simulink model "sgMdl_IO3xx_40_A2B_Loopback"  (R2024b)
settings: Solver=FixedStepAuto  StartTime=0.0  StopTime=inf  RelTol=1e-3  EnableMultiTasking=on
undefined symbols (not defined in the file): c, d, IO3xx, Pull, pull, up
libraries: speedgoatlib_a2b x6, simulink x3, speedgoatlib_interrupt x1, speedgoatlib_fpga x1
Description:
  | IO3xx A2B - Loopback
settings Model: ModifiedByFormat=Speedgoat  SimulationMode=external  ExtModeTrigDuration=100000  Creator=Speedgoat  LastModifiedBy=Speedgoat
settings SolverCC: ConcurrentTasks=on  AlgebraicLoopSolver=TrustRegion  PositivePriorityOrder=on  InsertRTBMode=Never (minimum delay)
settings DataIOCC: SaveFormat=Array  SaveState=on  SignalLoggingName=logsOut
settings OptimizationCC: BlockReduction=off  BooleanDataType=off  OptimizeBlockIOStorage=off  BufferReuse=off  GlobalBufferReuse=off  ExpressionFolding=off  LocalBlockOutputs=off  InitFltsAndDblsToZero=on  OptimizeDataStoreBuffers=off  BusAssignmentInplaceUpdate=off
settings DebuggingCC: SaveWithParameterizedLinksMsg=none  CheckExecutionContextPreStartOutputMsg=on  SignalResolutionControl=TryResolveAllWithWarning  TasksWithSamePriorityMsg=none  UnconnectedInputMsg=warning  UnconnectedOutputMsg=warning  UnconnectedLineMsg=warning  SFUnexpectedBacktrackingDiag=warning  SFNoUnconditionalDefaultTransitionDiag=warning  SFExecutionAtInitializationDiag=none  ArithmeticOperatorsInVariantConditions=warning
settings HardwareCC: ProdBitPerLong=64  ProdLongLongMode=on  ProdHWDeviceType=Intel->x86-64 (Linux 64)
settings ModelReferenceCC: EnableRefExpFcnMdlSchedulingChecks=on
settings SFSimCC: SimUseLocalCustomCode=off  SimTargetLang=C++
settings RTWCC: Description=Speedgoat Real-Time Target Machine  SystemTargetFile=speedgoat.tlc  TemplateMakefile=slrealtime_default_tmf  PostCodeGenCommand=sg.model.build.makeCfg(bdroot, buildInfo);  RTWUseLocalCustomCode=off  Toolchain=Simulink Real-Time Toolchain  BuildConfiguration=Faster Runs  TargetLang=C++  GPUComputeCapability=3.5  DLArmComputeVersion=19.05
settings CodeAppCC: StateflowObjectComments=on
settings SimulinkRealTimeTargetCC: SubcomponentCodeInterfacePackaging=Reusable function  MATLABClassNameForMDSCustomization=Simulink.SoftwareTarget.GRTCustomization  InstructionSetFMA=off  LogToMDFFile=off  SLRTFileLogMaxRuns=10  UseGCCFastMath=on
settings ConfigComp: CovMetricSettings=dw  CovSaveCumulativeToWorkspaceVar=on  CovSaveSingleToWorkspaceVar=on  CovExternalEMLEnable=off  CovSFcnEnable=off  CovBoundaryAbsTol=1.0e-5

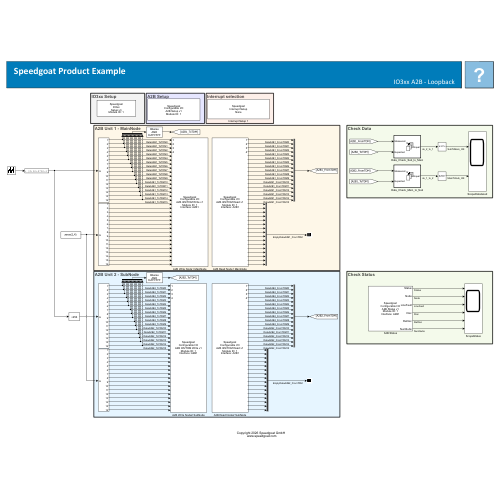
[thumbnail: Simulink's stored preview of the top-level diagram]
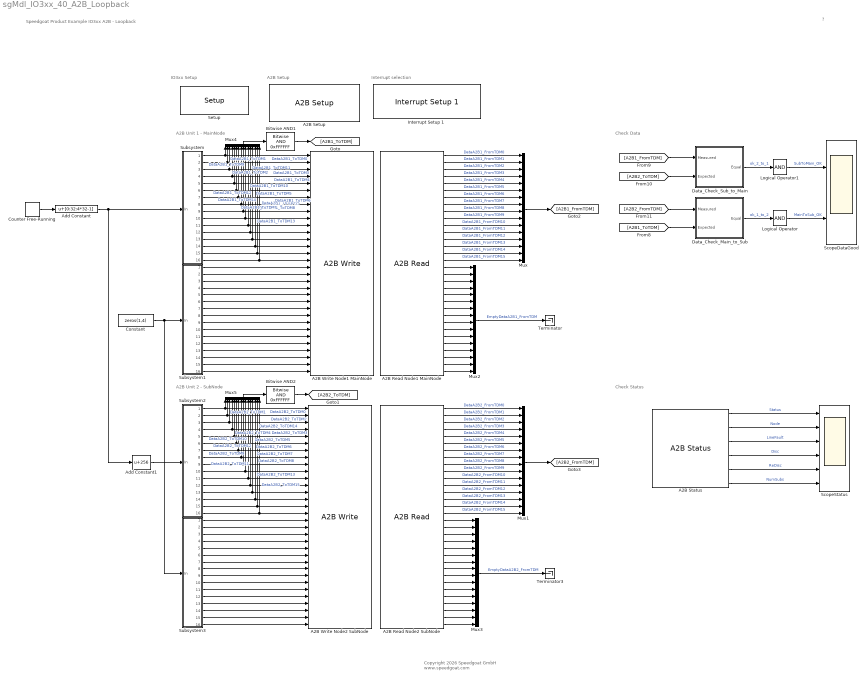
== system sgMdl_IO3xx_40_A2B_Loopback ==
  note: Interrupt selection
  note: A2B Setup
  note: IO3xx Setup
  note: A2B Unit 1 - MainNode
  note: A2B Unit 2 - SubNode
  note: Check Data
  note: Check Status
  note: Speedgoat Product Example
      | IO3xx A2B - Loopback
  note: ?
  note: Copyright 2026 Speedgoat GmbH
      |  www.speedgoat.com
  A2B Read Node1 MainNode : speedgoatlib_a2b/A2B Read   parModuleId=1  parPosition=A2B1  parFrameSize=4  parTdmMode=16  parTdmSize=32  parDataSize=24  parSampleTime=-1
  A2B Read Node2 SubNode : speedgoatlib_a2b/A2B Read   parModuleId=1  parPosition=A2B2  parFrameSize=4  parTdmMode=16  parTdmSize=32  parDataSize=24  parSampleTime=-1
  "A2B Setup " : speedgoatlib_a2b/A2B Setup   parModuleId=1  parPosition=1  parTdmChSize=[32 32 16 16]  parTdmMode=[16 16 0 0]  parA2BdownSlotSize=[24 0 0 0]  parA2BupSlotSize=[24 0 16 16]  parChecksum=2BC6806296FB9E7142791A9417BDFF8D,3D277645F3D52ECCF21C75D98A92E88D,c,d'  parMode1=Main Node  parMode2=Subordinate Node  parMode3=Disabled  parMode4=Disabled  parAudioClock=48kHz  parFrameSize=4  parSampleTime=4/48e3  parNetworkConfig1=''  parNodeConfig1=''  parNetworkConfig2=''  parNodeConfig2=''  parNetworkConfig3=''  parNodeConfig3=''  parNetworkConfig4=''  parNodeConfig4=''
  A2B Status : speedgoatlib_a2b/A2B Status   parModuleId=1  parChipId=A2B1  parEnPwr=on  parEnDiscovery=on  parEnBusDiscovery=on  parEnSlaveNodes=on  parSampleTime=50*4/48e3
  A2B Write Node1 MainNode : speedgoatlib_a2b/A2B Write   parModuleId=1  parPosition=A2B1  parFrameSize=4  parTdmMode=16  parTdmSize=32  parDataSize=24  parSampleTime=-1
  A2B Write Node2 SubNode : speedgoatlib_a2b/A2B Write   parModuleId=1  parPosition=A2B2  parFrameSize=4  parTdmMode=16  parTdmSize=32  parDataSize=24  parSampleTime=-1
  Add Constant : Bias  Bias=[0:32:4*32-1]  SaturateOnIntegerOverflow=off
  Add Constant1 : Bias  Bias=256  SaturateOnIntegerOverflow=off
  Bitwise AND1 : simulink/Logic and Bit Operations/Bitwise Operator  logicop=AND  UseBitMask=on  BitMask=0xFFFFFF  BitMaskRealWorld=Stored Integer
      settings: LibrarySourceBlock=|
      | simulink/Quick Insert/Logic and Bit
      | Operations/Bitwise AND
  Bitwise AND2 : simulink/Logic and Bit Operations/Bitwise Operator  logicop=AND  UseBitMask=on  BitMask=0xFFFFFF  BitMaskRealWorld=Stored Integer
      settings: LibrarySourceBlock=|
      | simulink/Quick Insert/Logic and Bit
      | Operations/Bitwise AND
  Constant : Constant  Value=zeros(1,4)  OutDataTypeStr=uint32
  Counter Free-Running : simulink/Sources/Counter Free-Running  NumBits=32  tsamp=-1
  Data_Check_Main_to_Sub : Subsystem  TreatAsAtomicUnit=on
  Data_Check_Sub_to_Main : Subsystem  TreatAsAtomicUnit=on
  Interrupt Setup 1 : speedgoatlib_interrupt/Interrupt Setup 1  parModuleTrigger=on  parPollingMode=on  parPriorityConf=High  parPriority=90  confStartFcn=IO324_200k_FPGA_POLLING_start_public  confStopFcn=IO324_200k_FPGA_POLLING_stop_public  confIsrFcn=IO324_200k_FPGA_POLLING_isr_public  confMapFcn=IO324_200k_FPGA_POLLING_map_public  confHookFile=io324_200k_fpga_polling_int_hooks.c  confIrqNr=-1  confIsPolling=on  confModID=16776961  confSelectedInt=None  confSelectedId=[]  confSelectedChannel=[]  confData=[90 1]  confForcePollingMode=off
  Logical Operator : Logic  Inputs=1  AllPortsSameDT=off  OutDataTypeStr=boolean
  Logical Operator1 : Logic  Inputs=1  AllPortsSameDT=off  OutDataTypeStr=boolean
  Mux{,1..5} (6 alike) : Mux  Inputs=16
  ScopeDataGood : Scope  NumInputPorts=2
  ScopeStatus : Scope  NumInputPorts=6
  Setup : speedgoatlib_fpga/Setup/Setup  board=Please select...  id=1  pciSlot=-1  device_id=1  bitstreamFilePath=[]  bitstreamFile=Please select...  fpgaFreq=100000000  enableDma=on  rearEnb_1=off  rearIO_1=IO3xx-40  rearEnb_2=off  rearIO_2=None  ProgSpiFlash=off  ProgBPIFlash=off  useFpgaDmaController=on  dmaTrigDropdown=Model Step  dmaTrigSelect=1  dmaStopOnOverload=on  dmaModeSequential=on  dmaModeParallel=off  PullRPort15=pull-up 3.3V  PullRPort31=pull-up 3.3V  PullRPort47=pull-up 3.3V  PullRPort63=pull-up 3.3V  diffLineTermination_1=on  diffLineTermination_2=on  diffLineTermination_3=on  diffLineTermination_4=on  diffLineTermination_5=on  diffLineTermination_6=on  diffLineTermination_7=on  diffLineTermination_8=on  diffLineTermination_9=on  diffLineTermination_10=on  diffLineTermination_11=on  diffLineTermination_12=on  diffLineTermination_13=on  diffLineTermination_14=on  diffLineTermination_15=on  diffLineTermination_16=on  diffLineTermination_17=on  diffLineTermination_18=on  diffLineTermination_19=on  diffLineTermination_20=on  diffLineTermination_21=on  diffLineTermination_22=on  diffLineTermination_23=on  diffLineTermination_24=on  diffLineTermination_25=on  diffLineTermination_26=on  diffLineTermination_27=on  diffLineTermination_28=on  diffLineTermination_29=on  diffLineTermination_30=on  diffLineTermination_31=on  diffLineTermination_32=on  ioVoltageDropDown1=3.3V  pullResistorDropDown1_1=Pull-up  pullResistorDropDown1_2=Pull-up  pullResistorDropDown1_3=Pull-up  pullResistorDropDown1_4=Pull-up  pullResistorDropDown1_5=Pull-up  pullResistorDropDown1_6=Pull-up  pullResistorDropDown1_7=Pull-up  pullResistorDropDown1_8=Pull-up  ttlIsImplementedCheckBox1=off  pullResistorDropDown2=Pull-up  ioVoltageDropDown2=3.3V  ttlIsImplementedCheckBox2=off  pullResistorDropDown3=Pull-up  ioVoltageDropDown3=3.3V  ttlIsImplementedCheckBox3=off  pullResistorDropDown4=Pull-up  ioVoltageDropDown4=3.3V  ttlIsImplementedCheckBox4=off  pullResistorDropDown5=Pull-up  ioVoltageDropDown5=3.3V  ttlIsImplementedCheckBox5=off  pullResistorDropDown6=Pull-up  ioVoltageDropDown6=3.3V  ttlIsImplementedCheckBox6=off  pullResistorDropDown7=Pull-up  ioVoltageDropDown7=3.3V  ttlIsImplementedCheckBox7=off  pullResistorDropDown8=Pull-up  ioVoltageDropDown8=3.3V  ttlIsImplementedCheckBox8=off  terminationCheckBox1=off  terminationCheckBox2=off  terminationCheckBox3=off  terminationCheckBox4=off  diffIsImplementedCheckBox1=off  terminationCheckBox5=off  terminationCheckBox6=off  terminationCheckBox7=off  terminationCheckBox8=off  diffIsImplementedCheckBox2=off  terminationCheckBox9=off  terminationCheckBox10=off  terminationCheckBox11=off  terminationCheckBox12=off  diffIsImplementedCheckBox3=off  terminationCheckBox13=off  terminationCheckBox14=off  terminationCheckBox15=off  terminationCheckBox16=off  diffIsImplementedCheckBox4=off  terminationCheckBox17=off  terminationCheckBox18=off  terminationCheckBox19=off  terminationCheckBox20=off  diffIsImplementedCheckBox5=off  terminationCheckBox21=off  terminationCheckBox22=off  terminationCheckBox23=off  terminationCheckBox24=off  diffIsImplementedCheckBox6=off  terminationCheckBox25=off  terminationCheckBox26=off  terminationCheckBox27=off  terminationCheckBox28=off  diffIsImplementedCheckBox7=off  terminationCheckBox29=off  terminationCheckBox30=off  terminationCheckBox31=off  terminationCheckBox32=off  diffIsImplementedCheckBox8=off  PullRPort0_1=pull-up  VioPort0_1=3.3V  PullRPort1_1=pull-up  VioPort1_1=3.3V  PullRPort2_1=pull-up  VioPort2_1=3.3V  PullRPort3_1=pull-up  VioPort3_1=3.3V  PullRPort4_1=pull-up  VioPort4_1=3.3V  PullRPort5_1=pull-up  VioPort5_1=3.3V  PullRPort6_1=pull-up  VioPort6_1=3.3V  diffLineTermination_rear1_1=on  diffLineTermination_rear1_2=on  diffLineTermination_rear1_3=on  diffLineTermination_rear1_4=on  diffLineTermination_rear1_5=on  diffLineTermination_rear1_6=on  diffLineTermination_rear1_7=on  diffLineTermination_rear1_8=on  PullRPort0_2=pull-up  VioPort0_2=3.3V  PullRPort1_2=pull-up  VioPort1_2=3.3V  PullRPort2_2=pull-up  VioPort2_2=3.3V  PullRPort3_2=pull-up  VioPort3_2=3.3V  PullRPort4_2=pull-up  VioPort4_2=3.3V  PullRPort5_2=pull-up  VioPort5_2=3.3V  PullRPort6_2=pull-up  VioPort6_2=3.3V  diffLineTermination_rear2_1=on  diffLineTermination_rear2_2=on  diffLineTermination_rear2_3=on  diffLineTermination_rear2_4=on  diffLineTermination_rear2_5=on  diffLineTermination_rear2_6=on  diffLineTermination_rear2_7=on  diffLineTermination_rear2_8=on
      settings: SourceProductName=IO3xx
  Subsystem : Subsystem
  Subsystem1 : Subsystem
  Subsystem2 : Subsystem
  Subsystem3 : Subsystem
  Terminator : Terminator
  Terminator3 : Terminator
  wires:
  A2B Read Node1 MainNode/19 -> Mux2/3
  Subsystem/4(Out4) -> A2B Write Node1 MainNode/4, Mux4/4  "DataA2B1_ToTDM3"
  Subsystem/16(Out16) -> A2B Write Node1 MainNode/16, Mux4/16  "DataA2B1_ToTDM15"
  Subsystem/9(Out9) -> A2B Write Node1 MainNode/9, Mux4/9  "DataA2B1_ToTDM8"
  A2B Read Node1 MainNode/16 -> Mux/16  "DataA2B1_FromTDM15"
  A2B Read Node1 MainNode/18 -> Mux2/2
  Subsystem/1(Out1) -> A2B Write Node1 MainNode/1, Mux4/1  "DataA2B1_ToTDM0"
  A2B Read Node1 MainNode/11 -> Mux/11  "DataA2B1_FromTDM10"
  A2B Read Node1 MainNode/31 -> Mux2/15
  Mux2/1 -> Terminator/1  "EmptyDataA2B1_FromTDM"
  Subsystem/12(Out12) -> A2B Write Node1 MainNode/12, Mux4/12  "DataA2B1_ToTDM11"
  A2B Read Node1 MainNode/22 -> Mux2/6
  A2B Read Node1 MainNode/9 -> Mux/9  "DataA2B1_FromTDM8"
  A2B Read Node1 MainNode/12 -> Mux/12  "DataA2B1_FromTDM11"
  Subsystem/11(Out11) -> A2B Write Node1 MainNode/11, Mux4/11  "DataA2B1_ToTDM10"
  Subsystem/6(Out6) -> A2B Write Node1 MainNode/6, Mux4/6  "DataA2B1_ToTDM5"
  Subsystem/14(Out14) -> A2B Write Node1 MainNode/14, Mux4/14  "DataA2B1_ToTDM13"
  A2B Read Node1 MainNode/32 -> Mux2/16
  Subsystem/15(Out15) -> A2B Write Node1 MainNode/15, Mux4/15  "DataA2B1_ToTDM14"
  A2B Read Node1 MainNode/24 -> Mux2/8
  A2B Read Node1 MainNode/30 -> Mux2/14
  Mux/1 -> [A2B1_FromTDM]
  A2B Read Node1 MainNode/5 -> Mux/5  "DataA2B1_FromTDM4"
  A2B Read Node1 MainNode/25 -> Mux2/9
  Subsystem/7(Out7) -> A2B Write Node1 MainNode/7, Mux4/7  "DataA2B1_ToTDM6"
  A2B Read Node1 MainNode/4 -> Mux/4  "DataA2B1_FromTDM3"
  A2B Read Node1 MainNode/13 -> Mux/13  "DataA2B1_FromTDM12"
  A2B Read Node1 MainNode/8 -> Mux/8  "DataA2B1_FromTDM7"
  A2B Read Node1 MainNode/3 -> Mux/3  "DataA2B1_FromTDM2"
  A2B Read Node1 MainNode/6 -> Mux/6  "DataA2B1_FromTDM5"
  A2B Read Node1 MainNode/27 -> Mux2/11
  Subsystem/8(Out8) -> A2B Write Node1 MainNode/8, Mux4/8  "DataA2B1_ToTDM7"
  A2B Read Node1 MainNode/26 -> Mux2/10
  A2B Read Node1 MainNode/2 -> Mux/2  "DataA2B1_FromTDM1"
  A2B Read Node1 MainNode/17 -> Mux2/1
  Subsystem/13(Out13) -> A2B Write Node1 MainNode/13, Mux4/13  "DataA2B1_ToTDM12"
  A2B Read Node1 MainNode/14 -> Mux/14  "DataA2B1_FromTDM13"
  A2B Read Node1 MainNode/23 -> Mux2/7
  Subsystem/5(Out5) -> A2B Write Node1 MainNode/5, Mux4/5  "DataA2B1_ToTDM4"
  A2B Read Node1 MainNode/10 -> Mux/10  "DataA2B1_FromTDM9"
  A2B Read Node1 MainNode/7 -> Mux/7  "DataA2B1_FromTDM6"
  A2B Read Node1 MainNode/21 -> Mux2/5
  A2B Read Node1 MainNode/1 -> Mux/1  "DataA2B1_FromTDM0"
  A2B Read Node1 MainNode/29 -> Mux2/13
  A2B Read Node1 MainNode/20 -> Mux2/4
  A2B Read Node1 MainNode/28 -> Mux2/12
  Subsystem/10(Out10) -> A2B Write Node1 MainNode/10, Mux4/10  "DataA2B1_ToTDM9"
  A2B Read Node1 MainNode/15 -> Mux/15  "DataA2B1_FromTDM14"
  A2B Read Node2 SubNode/25 -> Mux3/9
  A2B Read Node2 SubNode/24 -> Mux3/8
  A2B Read Node2 SubNode/28 -> Mux3/12
  A2B Read Node2 SubNode/18 -> Mux3/2
  A2B Read Node2 SubNode/19 -> Mux3/3
  Subsystem3/9(Out9) -> A2B Write Node2 SubNode/25
  Subsystem3/14(Out14) -> A2B Write Node2 SubNode/30
  A2B Read Node2 SubNode/27 -> Mux3/11
  A2B Read Node2 SubNode/29 -> Mux3/13
  A2B Read Node2 SubNode/26 -> Mux3/10
  A2B Read Node2 SubNode/31 -> Mux3/15
  Subsystem3/8(Out8) -> A2B Write Node2 SubNode/24
  A2B Read Node2 SubNode/30 -> Mux3/14
  Mux3/1 -> Terminator3/1  "EmptyDataA2B2_FromTDM"
  Subsystem3/13(Out13) -> A2B Write Node2 SubNode/29
  Subsystem3/7(Out7) -> A2B Write Node2 SubNode/23
  A2B Read Node2 SubNode/20 -> Mux3/4
  A2B Read Node2 SubNode/17 -> Mux3/1
  A2B Read Node2 SubNode/32 -> Mux3/16
  Subsystem3/10(Out10) -> A2B Write Node2 SubNode/26
  A2B Read Node2 SubNode/23 -> Mux3/7
  Subsystem3/12(Out12) -> A2B Write Node2 SubNode/28
  Subsystem3/5(Out5) -> A2B Write Node2 SubNode/21
  Subsystem3/3(Out3) -> A2B Write Node2 SubNode/19
  Subsystem3/11(Out11) -> A2B Write Node2 SubNode/27
  Subsystem3/6(Out6) -> A2B Write Node2 SubNode/22
  Subsystem3/16(Out16) -> A2B Write Node2 SubNode/32
  A2B Read Node2 SubNode/22 -> Mux3/6
  Subsystem3/4(Out4) -> A2B Write Node2 SubNode/20
  Subsystem3/2(Out2) -> A2B Write Node2 SubNode/18
  A2B Read Node2 SubNode/21 -> Mux3/5
  Subsystem3/15(Out15) -> A2B Write Node2 SubNode/31
  Subsystem/3(Out3) -> A2B Write Node1 MainNode/3, Mux4/3  "DataA2B1_ToTDM2"
  Subsystem1/1(Out1) -> A2B Write Node1 MainNode/17
  Subsystem1/2(Out2) -> A2B Write Node1 MainNode/18
  Subsystem1/3(Out3) -> A2B Write Node1 MainNode/19
  Subsystem1/4(Out4) -> A2B Write Node1 MainNode/20
  Subsystem1/5(Out5) -> A2B Write Node1 MainNode/21
  Subsystem1/6(Out6) -> A2B Write Node1 MainNode/22
  Subsystem1/7(Out7) -> A2B Write Node1 MainNode/23
  Subsystem1/8(Out8) -> A2B Write Node1 MainNode/24
  Subsystem1/9(Out9) -> A2B Write Node1 MainNode/25
  Subsystem1/10(Out10) -> A2B Write Node1 MainNode/26
  Subsystem1/11(Out11) -> A2B Write Node1 MainNode/27
  Subsystem1/12(Out12) -> A2B Write Node1 MainNode/28
  Subsystem1/13(Out13) -> A2B Write Node1 MainNode/29
  Subsystem1/14(Out14) -> A2B Write Node1 MainNode/30
  Subsystem1/15(Out15) -> A2B Write Node1 MainNode/31
  Subsystem1/16(Out16) -> A2B Write Node1 MainNode/32
  Add Constant/1 -> Add Constant1/1, Subsystem/1(In)
  Counter Free-Running/1 -> Add Constant/1
  Add Constant1/1 -> Subsystem2/1(In)
  Constant/1 -> Subsystem1/1(In), Subsystem3/1(In)
  [A2B1_ToTDM] -> Data_Check_Main_to_Sub/2(Expected)
  [A2B1_FromTDM] -> Data_Check_Sub_to_Main/1(Measured)
  Data_Check_Main_to_Sub/1(Equal) -> Logical Operator/1  "ok_1_to_2"
  [A2B2_FromTDM] -> Data_Check_Main_to_Sub/1(Measured)
  Logical Operator1/1 -> ScopeDataGood/1  "SubToMain_OK"
  Data_Check_Sub_to_Main/1(Equal) -> Logical Operator1/1  "ok_2_to_1"
  [A2B2_ToTDM] -> Data_Check_Sub_to_Main/2(Expected)
  Logical Operator/1 -> ScopeDataGood/2  "MainToSub_OK"
  A2B Status/3 -> ScopeStatus/3  "LineFault"
  A2B Status/5 -> ScopeStatus/5  "ReDisc"
  A2B Status/4 -> ScopeStatus/4  "Disc"
  A2B Status/6 -> ScopeStatus/6  "NumSubs"
  A2B Status/1 -> ScopeStatus/1  "Status"
  A2B Status/2 -> ScopeStatus/2  "Node"
  Subsystem/2(Out2) -> Mux4/2, A2B Write Node1 MainNode/2  "DataA2B1_ToTDM1"
  A2B Read Node2 SubNode/15 -> Mux1/15  "DataA2B2_FromTDM14"
  A2B Read Node2 SubNode/1 -> Mux1/1  "DataA2B2_FromTDM0"
  A2B Read Node2 SubNode/7 -> Mux1/7  "DataA2B2_FromTDM6"
  A2B Read Node2 SubNode/10 -> Mux1/10  "DataA2B2_FromTDM9"
  A2B Read Node2 SubNode/14 -> Mux1/14  "DataA2B2_FromTDM13"
  A2B Read Node2 SubNode/2 -> Mux1/2  "DataA2B2_FromTDM1"
  A2B Read Node2 SubNode/6 -> Mux1/6  "DataA2B2_FromTDM5"
  A2B Read Node2 SubNode/3 -> Mux1/3  "DataA2B2_FromTDM2"
  A2B Read Node2 SubNode/8 -> Mux1/8  "DataA2B2_FromTDM7"
  A2B Read Node2 SubNode/13 -> Mux1/13  "DataA2B2_FromTDM12"
  A2B Read Node2 SubNode/4 -> Mux1/4  "DataA2B2_FromTDM3"
  A2B Read Node2 SubNode/5 -> Mux1/5  "DataA2B2_FromTDM4"
  Mux1/1 -> [A2B2_FromTDM]
  A2B Read Node2 SubNode/12 -> Mux1/12  "DataA2B2_FromTDM11"
  A2B Read Node2 SubNode/9 -> Mux1/9  "DataA2B2_FromTDM8"
  A2B Read Node2 SubNode/11 -> Mux1/11  "DataA2B2_FromTDM10"
  A2B Read Node2 SubNode/16 -> Mux1/16  "DataA2B2_FromTDM15"
  Subsystem2/6(Out6) -> A2B Write Node2 SubNode/6, Mux5/6  "DataA2B2_ToTDM5"
  Subsystem2/8(Out8) -> A2B Write Node2 SubNode/8, Mux5/8  "DataA2B2_ToTDM7"
  Subsystem2/1(Out1) -> A2B Write Node2 SubNode/1, Mux5/1  "DataA2B2_ToTDM0"
  Subsystem2/14(Out14) -> A2B Write Node2 SubNode/14, Mux5/14  "DataA2B2_ToTDM13"
  Subsystem2/7(Out7) -> A2B Write Node2 SubNode/7, Mux5/7  "DataA2B2_ToTDM6"
  Subsystem2/15(Out15) -> A2B Write Node2 SubNode/15, Mux5/15  "DataA2B2_ToTDM14"
  Subsystem2/9(Out9) -> A2B Write Node2 SubNode/9, Mux5/9  "DataA2B2_ToTDM8"
  Subsystem2/13(Out13) -> A2B Write Node2 SubNode/13, Mux5/13  "DataA2B2_ToTDM12"
  Subsystem2/4(Out4) -> A2B Write Node2 SubNode/4, Mux5/4  "DataA2B2_ToTDM3"
  Subsystem2/3(Out3) -> A2B Write Node2 SubNode/3, Mux5/3  "DataA2B2_ToTDM2"
  Subsystem2/2(Out2) -> A2B Write Node2 SubNode/2, Mux5/2  "DataA2B2_ToTDM1"
  Subsystem2/10(Out10) -> A2B Write Node2 SubNode/10, Mux5/10  "DataA2B2_ToTDM9"
  Subsystem2/11(Out11) -> A2B Write Node2 SubNode/11, Mux5/11  "DataA2B2_ToTDM10"
  Subsystem2/16(Out16) -> A2B Write Node2 SubNode/16, Mux5/16  "DataA2B2_ToTDM15"
  Subsystem2/5(Out5) -> A2B Write Node2 SubNode/5, Mux5/5  "DataA2B2_ToTDM4"
  Subsystem2/12(Out12) -> A2B Write Node2 SubNode/12, Mux5/12  "DataA2B2_ToTDM11"
  Subsystem3/1(Out1) -> A2B Write Node2 SubNode/17
  Mux5/1 -> Bitwise AND2/1
  Mux4/1 -> Bitwise AND1/1
  Bitwise AND1/1 -> [A2B1_ToTDM]
  Bitwise AND2/1 -> [A2B2_ToTDM]

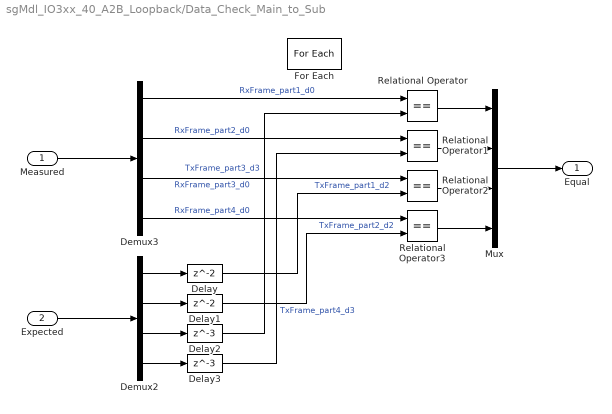
== system sgMdl_IO3xx_40_A2B_Loopback/Data_Check_Main_to_Sub ==
  Measured : Inport  Partition=on  PartitionDimension=1  PartitionWidth=4  PartitionOffset=0
  Expected : Inport  Port=2  Partition=on  PartitionDimension=1  PartitionWidth=4  PartitionOffset=0
  Delay : Delay
  Delay1 : Delay
  Delay2 : Delay  DelayLength=3
  Delay3 : Delay  DelayLength=3
  Demux2 : Demux
  Demux3 : Demux
  For Each : ForEach  DisableCoverage=on
  Mux : Mux
  Relational Operator{,1..3} (4 alike) : RelationalOperator  Operator===  OutDataTypeStr=boolean  RndMeth=Simplest  InputSameDT=off
  Equal : Outport  ConcatenationDimension=1
  wires:
  Delay3/1 -> Relational Operator1/2  "TxFrame_part4_d3"
  Delay2/1 -> Relational Operator/2  "TxFrame_part3_d3"
  Delay1/1 -> Relational Operator3/2  "TxFrame_part2_d2"
  Delay/1 -> Relational Operator2/2  "TxFrame_part1_d2"
  Demux3/1 -> Relational Operator/1  "RxFrame_part1_d0"
  Demux3/2 -> Relational Operator1/1  "RxFrame_part2_d0"
  Demux3/3 -> Relational Operator2/1  "RxFrame_part3_d0"
  Demux3/4 -> Relational Operator3/1  "RxFrame_part4_d0"
  Demux2/1 -> Delay/1
  Demux2/3 -> Delay2/1
  Demux2/2 -> Delay1/1
  Demux2/4 -> Delay3/1
  Expected/1 -> Demux2/1
  Measured/1 -> Demux3/1
  Relational Operator/1 -> Mux/1
  Relational Operator1/1 -> Mux/2
  Relational Operator2/1 -> Mux/3
  Relational Operator3/1 -> Mux/4
  Mux/1 -> Equal/1

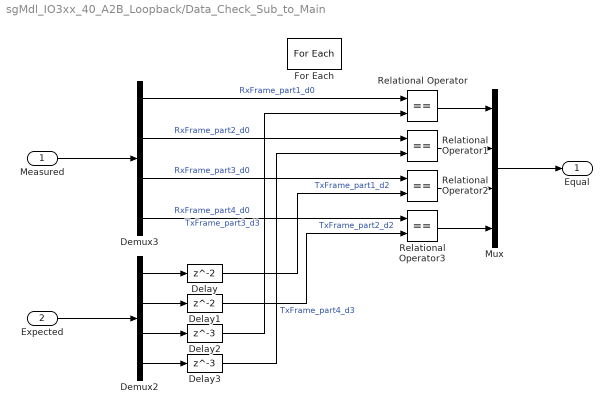
== system sgMdl_IO3xx_40_A2B_Loopback/Data_Check_Sub_to_Main ==
  Measured : Inport  Partition=on  PartitionDimension=1  PartitionWidth=4  PartitionOffset=0
  Expected : Inport  Port=2  Partition=on  PartitionDimension=1  PartitionWidth=4  PartitionOffset=0
  Delay : Delay
  Delay1 : Delay
  Delay2 : Delay  DelayLength=3
  Delay3 : Delay  DelayLength=3
  Demux2 : Demux
  Demux3 : Demux
  For Each : ForEach  DisableCoverage=on
  Mux : Mux
  Relational Operator{,1..3} (4 alike) : RelationalOperator  Operator===  OutDataTypeStr=boolean  RndMeth=Simplest  InputSameDT=off
  Equal : Outport  ConcatenationDimension=1
  wires:
  Mux/1 -> Equal/1
  Relational Operator3/1 -> Mux/4
  Relational Operator2/1 -> Mux/3
  Relational Operator1/1 -> Mux/2
  Relational Operator/1 -> Mux/1
  Measured/1 -> Demux3/1
  Expected/1 -> Demux2/1
  Demux2/4 -> Delay3/1
  Demux2/2 -> Delay1/1
  Demux2/3 -> Delay2/1
  Demux2/1 -> Delay/1
  Demux3/4 -> Relational Operator3/1  "RxFrame_part4_d0"
  Demux3/3 -> Relational Operator2/1  "RxFrame_part3_d0"
  Demux3/2 -> Relational Operator1/1  "RxFrame_part2_d0"
  Demux3/1 -> Relational Operator/1  "RxFrame_part1_d0"
  Delay/1 -> Relational Operator2/2  "TxFrame_part1_d2"
  Delay1/1 -> Relational Operator3/2  "TxFrame_part2_d2"
  Delay2/1 -> Relational Operator/2  "TxFrame_part3_d3"
  Delay3/1 -> Relational Operator1/2  "TxFrame_part4_d3"

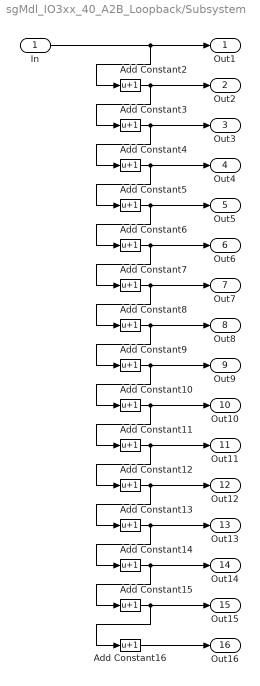
== system sgMdl_IO3xx_40_A2B_Loopback/Subsystem ==
  In : Inport
  Add Constant{2..16} (15 alike) : Bias  Bias=1  SaturateOnIntegerOverflow=off
  Out1 : Outport
  Out2 : Outport  Port=2
  Out3 : Outport  Port=3
  Out4 : Outport  Port=4
  Out5 : Outport  Port=5
  Out6 : Outport  Port=6
  Out7 : Outport  Port=7
  Out8 : Outport  Port=8
  Out9 : Outport  Port=9
  Out10 : Outport  Port=10
  Out11 : Outport  Port=11
  Out12 : Outport  Port=12
  Out13 : Outport  Port=13
  Out14 : Outport  Port=14
  Out15 : Outport  Port=15
  Out16 : Outport  Port=16
  wires:
  In/1 -> Out1/1, Add Constant2/1
  Add Constant2/1 -> Out2/1, Add Constant3/1
  Add Constant4/1 -> Out4/1, Add Constant5/1
  Add Constant3/1 -> Out3/1, Add Constant4/1
  Add Constant7/1 -> Out7/1, Add Constant8/1
  Add Constant8/1 -> Out8/1, Add Constant9/1
  Add Constant6/1 -> Out6/1, Add Constant7/1
  Add Constant5/1 -> Out5/1, Add Constant6/1
  Add Constant13/1 -> Out13/1, Add Constant14/1
  Add Constant14/1 -> Out14/1, Add Constant15/1
  Add Constant16/1 -> Out16/1
  Add Constant15/1 -> Out15/1, Add Constant16/1
  Add Constant11/1 -> Out11/1, Add Constant12/1
  Add Constant12/1 -> Out12/1, Add Constant13/1
  Add Constant10/1 -> Out10/1, Add Constant11/1
  Add Constant9/1 -> Out9/1, Add Constant10/1

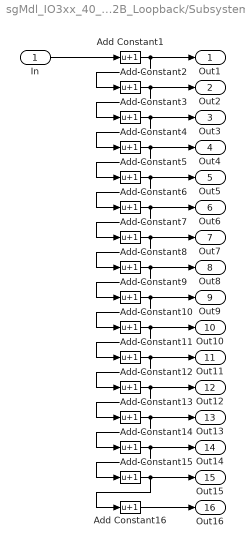
== system sgMdl_IO3xx_40_A2B_Loopback/Subsystem1 ==
  In : Inport
  Add Constant{1..16} (16 alike) : Bias  Bias=1  SaturateOnIntegerOverflow=off
  Out1 : Outport
  Out2 : Outport  Port=2
  Out3 : Outport  Port=3
  Out4 : Outport  Port=4
  Out5 : Outport  Port=5
  Out6 : Outport  Port=6
  Out7 : Outport  Port=7
  Out8 : Outport  Port=8
  Out9 : Outport  Port=9
  Out10 : Outport  Port=10
  Out11 : Outport  Port=11
  Out12 : Outport  Port=12
  Out13 : Outport  Port=13
  Out14 : Outport  Port=14
  Out15 : Outport  Port=15
  Out16 : Outport  Port=16
  wires:
  Add Constant9/1 -> Add Constant10/1, Out9/1
  Add Constant10/1 -> Add Constant11/1, Out10/1
  Add Constant12/1 -> Add Constant13/1, Out12/1
  Add Constant11/1 -> Out11/1, Add Constant12/1
  Add Constant15/1 -> Add Constant16/1, Out15/1
  Add Constant16/1 -> Out16/1
  Add Constant14/1 -> Out14/1, Add Constant15/1
  Add Constant13/1 -> Out13/1, Add Constant14/1
  Add Constant5/1 -> Add Constant6/1, Out5/1
  Add Constant6/1 -> Add Constant7/1, Out6/1
  Add Constant8/1 -> Out8/1, Add Constant9/1
  Add Constant7/1 -> Out7/1, Add Constant8/1
  Add Constant3/1 -> Add Constant4/1, Out3/1
  Add Constant4/1 -> Out4/1, Add Constant5/1
  Add Constant2/1 -> Out2/1, Add Constant3/1
  Add Constant1/1 -> Out1/1, Add Constant2/1
  In/1 -> Add Constant1/1

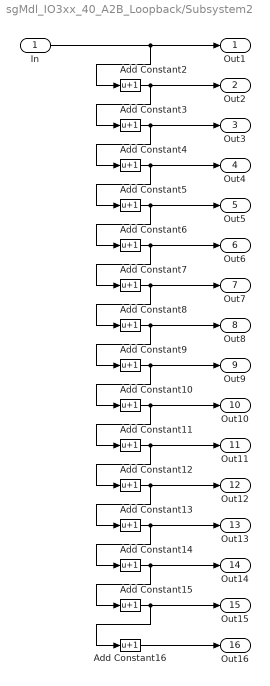
== system sgMdl_IO3xx_40_A2B_Loopback/Subsystem2 ==
  In : Inport
  Add Constant{2..16} (15 alike) : Bias  Bias=1  SaturateOnIntegerOverflow=off
  Out1 : Outport
  Out2 : Outport  Port=2
  Out3 : Outport  Port=3
  Out4 : Outport  Port=4
  Out5 : Outport  Port=5
  Out6 : Outport  Port=6
  Out7 : Outport  Port=7
  Out8 : Outport  Port=8
  Out9 : Outport  Port=9
  Out10 : Outport  Port=10
  Out11 : Outport  Port=11
  Out12 : Outport  Port=12
  Out13 : Outport  Port=13
  Out14 : Outport  Port=14
  Out15 : Outport  Port=15
  Out16 : Outport  Port=16
  wires:
  Add Constant9/1 -> Out9/1, Add Constant10/1
  Add Constant10/1 -> Out10/1, Add Constant11/1
  Add Constant12/1 -> Out12/1, Add Constant13/1
  Add Constant11/1 -> Out11/1, Add Constant12/1
  Add Constant15/1 -> Out15/1, Add Constant16/1
  Add Constant16/1 -> Out16/1
  Add Constant14/1 -> Out14/1, Add Constant15/1
  Add Constant13/1 -> Out13/1, Add Constant14/1
  Add Constant5/1 -> Out5/1, Add Constant6/1
  Add Constant6/1 -> Out6/1, Add Constant7/1
  Add Constant8/1 -> Out8/1, Add Constant9/1
  Add Constant7/1 -> Out7/1, Add Constant8/1
  Add Constant3/1 -> Out3/1, Add Constant4/1
  Add Constant4/1 -> Out4/1, Add Constant5/1
  Add Constant2/1 -> Out2/1, Add Constant3/1
  In/1 -> Out1/1, Add Constant2/1

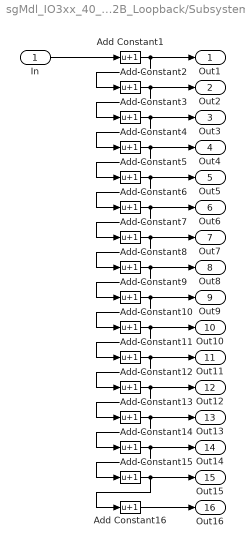
== system sgMdl_IO3xx_40_A2B_Loopback/Subsystem3 ==
  In : Inport
  Add Constant{1..16} (16 alike) : Bias  Bias=1  SaturateOnIntegerOverflow=off
  Out1 : Outport
  Out2 : Outport  Port=2
  Out3 : Outport  Port=3
  Out4 : Outport  Port=4
  Out5 : Outport  Port=5
  Out6 : Outport  Port=6
  Out7 : Outport  Port=7
  Out8 : Outport  Port=8
  Out9 : Outport  Port=9
  Out10 : Outport  Port=10
  Out11 : Outport  Port=11
  Out12 : Outport  Port=12
  Out13 : Outport  Port=13
  Out14 : Outport  Port=14
  Out15 : Outport  Port=15
  Out16 : Outport  Port=16
  wires:
  In/1 -> Add Constant1/1
  Add Constant1/1 -> Add Constant2/1, Out1/1
  Add Constant2/1 -> Add Constant3/1, Out2/1
  Add Constant4/1 -> Add Constant5/1, Out4/1
  Add Constant3/1 -> Out3/1, Add Constant4/1
  Add Constant7/1 -> Add Constant8/1, Out7/1
  Add Constant8/1 -> Add Constant9/1, Out8/1
  Add Constant6/1 -> Out6/1, Add Constant7/1
  Add Constant5/1 -> Out5/1, Add Constant6/1
  Add Constant13/1 -> Add Constant14/1, Out13/1
  Add Constant14/1 -> Add Constant15/1, Out14/1
  Add Constant16/1 -> Out16/1
  Add Constant15/1 -> Out15/1, Add Constant16/1
  Add Constant11/1 -> Add Constant12/1, Out11/1
  Add Constant12/1 -> Out12/1, Add Constant13/1
  Add Constant10/1 -> Out10/1, Add Constant11/1
  Add Constant9/1 -> Out9/1, Add Constant10/1
